simulink model "RLModel"  (R2024b)
settings: Solver=VariableStepAuto  StartTime=0.0  StopTime=Tf  RelTol=1e-3  AbsTol=1e-3  EnableMultiTasking=on
InitFcn:
  | ModelParameters;
values from neighbouring files (symbols this model uses):
  foot_height = 0.05    [ModelParameters.m]
  foot_length = 0.3    [ModelParameters.m]
  foot_width = 0.2    [ModelParameters.m]
  init_height = plane_height/2 + foot_height + shank_height + thigh_height + 0.5*torso_height    (= 1.65)    [ModelParameters.m]
  max_torque = 1000    [ModelParameters.m]
  plane_height = 0.2    [ModelParameters.m]
  shank_height = 0.5    [ModelParameters.m]
  shank_length = 0.2    [ModelParameters.m]
  shank_width = 0.2    [ModelParameters.m]
  thigh_height = 0.5    [ModelParameters.m]
  thigh_length = 0.2    [ModelParameters.m]
  thigh_width = 0.2    [ModelParameters.m]
  torso_height = 1.0    (= 1)    [ModelParameters.m]
  torso_length = 0.2    [ModelParameters.m]
  torso_width = 0.5    [ModelParameters.m]
undefined symbols (not defined in the file or in its folder): X, Y, Z
libraries: sm_lib x53, nesl_utility x32, simulink x2, rllib x1, aerolibconvert2 x1
(part 3 of 3)

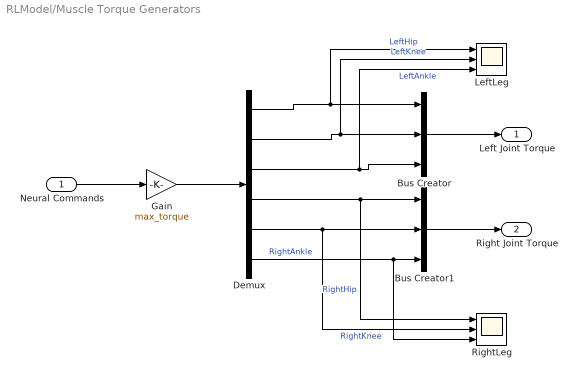
== system RLModel/Muscle Torque Generators ==
  Neural Commands : Inport
  Bus Creator : BusCreator  Inputs=3
  Bus Creator1 : BusCreator  Inputs=3
  Demux : Demux  Outputs=6
  Gain : Gain  Gain=max_torque
  LeftLeg : Scope  NumInputPorts=3
  RightLeg : Scope  NumInputPorts=3
  Left Joint Torque : Outport
  Right Joint Torque : Outport  Port=2
  wires:
  Demux/1 -> LeftLeg/1, Bus Creator/1  "LeftHip"
  Bus Creator/1 -> Left Joint Torque/1
  Bus Creator1/1 -> Right Joint Torque/1
  Demux/2 -> LeftLeg/2, Bus Creator/2  "LeftKnee"
  Demux/3 -> LeftLeg/3, Bus Creator/3  "LeftAnkle"
  Demux/4 -> RightLeg/1, Bus Creator1/1  "RightHip"
  Demux/5 -> Bus Creator1/2, RightLeg/2  "RightKnee"
  Demux/6 -> RightLeg/3, Bus Creator1/3  "RightAnkle"
  Neural Commands/1 -> Gain/1
  Gain/1 -> Demux/1

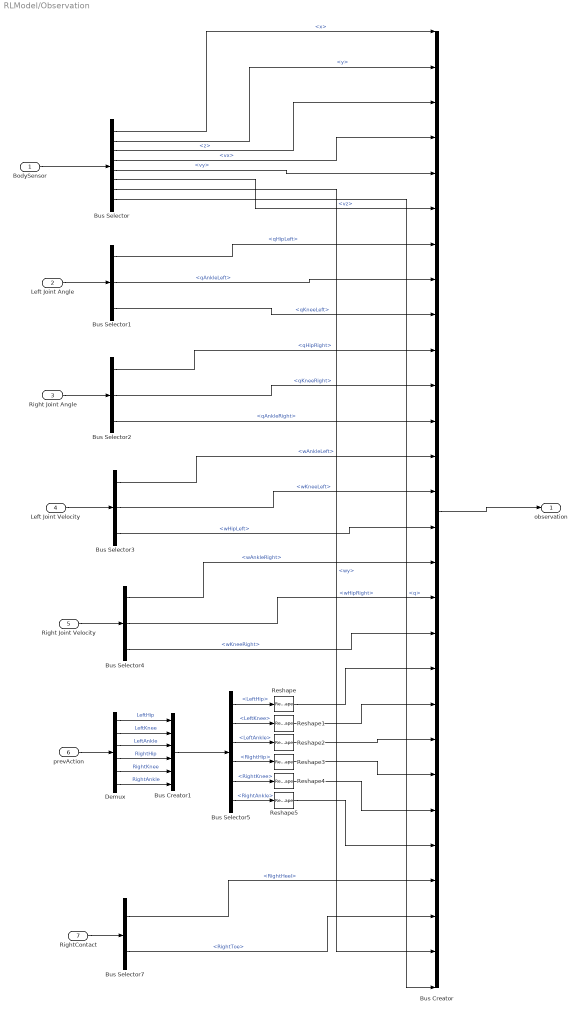
== system RLModel/Observation ==
  BodySensor : Inport
  Left Joint Angle : Inport  Port=2
  Right Joint Angle : Inport  Port=3
  Left Joint Velocity : Inport  Port=4
  Right Joint Velocity : Inport  Port=5
  prevAction : Inport  Port=6
  RightContact : Inport  Port=7
  Bus Creator : BusCreator  Inputs=28
  Bus Creator1 : BusCreator  Inputs=6
  Bus Selector : BusSelector  OutputSignals=x,y,z,vx,vy,vz,wy,q
  Bus Selector1 : BusSelector  OutputSignals=qHipLeft,qAnkleLeft,qKneeLeft
  Bus Selector2 : BusSelector  OutputSignals=qHipRight,qKneeRight,qAnkleRight
  Bus Selector3 : BusSelector  OutputSignals=wAnkleLeft,wKneeLeft,wHipLeft
  Bus Selector4 : BusSelector  OutputSignals=wAnkleRight,wHipRight,wKneeRight
  Bus Selector5 : BusSelector  OutputSignals=LeftHip,LeftKnee,LeftAnkle,RightHip,RightKnee,RightAnkle
  Bus Selector7 : BusSelector  OutputSignals=RightHeel,RightToe
  Demux : Demux  Outputs=6
  Reshape{,1..5} (6 alike) : Reshape  OutputDimensionality=Customize  OutputDimensions=1
  observation : Outport
  wires:
  BodySensor/1 -> Bus Selector/1
  Left Joint Angle/1 -> Bus Selector1/1
  Right Joint Angle/1 -> Bus Selector2/1
  Left Joint Velocity/1 -> Bus Selector3/1
  Right Joint Velocity/1 -> Bus Selector4/1
  Bus Selector/1 -> Bus Creator/1  "<x>"
  Bus Selector/2 -> Bus Creator/2  "<y>"
  Bus Selector/3 -> Bus Creator/3  "<z>"
  Bus Selector/4 -> Bus Creator/4  "<vx>"
  Bus Selector/5 -> Bus Creator/5  "<vy>"
  Bus Selector/6 -> Bus Creator/6  "<vz>"
  Bus Selector1/1 -> Bus Creator/7  "<qHipLeft>"
  Bus Selector1/2 -> Bus Creator/8  "<qAnkleLeft>"
  Bus Selector1/3 -> Bus Creator/9  "<qKneeLeft>"
  Bus Selector2/1 -> Bus Creator/10  "<qHipRight>"
  Bus Selector2/2 -> Bus Creator/11  "<qKneeRight>"
  Bus Selector2/3 -> Bus Creator/12  "<qAnkleRight>"
  Bus Selector3/1 -> Bus Creator/13  "<wAnkleLeft>"
  Bus Selector3/2 -> Bus Creator/14  "<wKneeLeft>"
  Bus Selector3/3 -> Bus Creator/15  "<wHipLeft>"
  Bus Selector4/1 -> Bus Creator/16  "<wAnkleRight>"
  Bus Selector4/2 -> Bus Creator/17  "<wHipRight>"
  Bus Selector4/3 -> Bus Creator/18  "<wKneeRight>"
  Bus Creator/1 -> observation/1
  prevAction/1 -> Demux/1
  Demux/1 -> Bus Creator1/1  "LeftHip"
  Demux/2 -> Bus Creator1/2  "LeftKnee"
  Demux/3 -> Bus Creator1/3  "LeftAnkle"
  Demux/4 -> Bus Creator1/4  "RightHip"
  Demux/5 -> Bus Creator1/5  "RightKnee"
  Demux/6 -> Bus Creator1/6  "RightAnkle"
  Bus Creator1/1 -> Bus Selector5/1
  Bus Selector5/1 -> Reshape/1  "<LeftHip>"
  Reshape/1 -> Bus Creator/19
  Bus Selector5/2 -> Reshape1/1  "<LeftKnee>"
  Bus Selector5/3 -> Reshape2/1  "<LeftAnkle>"
  Bus Selector5/4 -> Reshape3/1  "<RightHip>"
  Bus Selector5/5 -> Reshape4/1  "<RightKnee>"
  Bus Selector5/6 -> Reshape5/1  "<RightAnkle>"
  Reshape1/1 -> Bus Creator/20
  Reshape2/1 -> Bus Creator/21
  Reshape3/1 -> Bus Creator/22
  Reshape4/1 -> Bus Creator/23
  Reshape5/1 -> Bus Creator/24
  RightContact/1 -> Bus Selector7/1
  Bus Selector7/1 -> Bus Creator/25  "<RightHeel>"
  Bus Selector7/2 -> Bus Creator/26  "<RightToe>"
  Bus Selector/7 -> Bus Creator/27  "<wy>"
  Bus Selector/8 -> Bus Creator/28  "<q>"

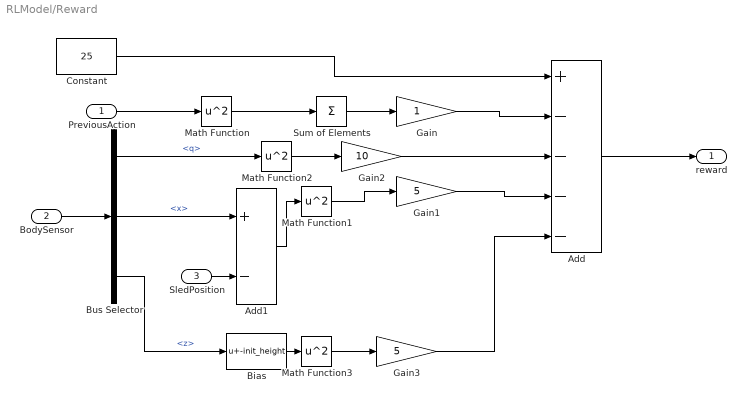
== system RLModel/Reward ==
  PreviousAction : Inport
  BodySensor : Inport  Port=2
  SledPosition : Inport  Port=3
  Add : Sum  Inputs=+----
  Add1 : Sum  Inputs=+-
  Bias : Bias  Bias=-init_height  SaturateOnIntegerOverflow=off
  Bus Selector : BusSelector  OutputSignals=q,x,z
  Constant : Constant  Value=25
  Gain : Gain
  Gain1 : Gain  Gain=5
  Gain2 : Gain  Gain=10
  Gain3 : Gain  Gain=5
  Math Function{,1..3} (4 alike) : Math  Operator=square
  Sum of Elements : Sum  Inputs=+
  reward : Outport
  wires:
  PreviousAction/1 -> Math Function/1
  Math Function/1 -> Sum of Elements/1
  Sum of Elements/1 -> Gain/1
  Add/1 -> reward/1
  BodySensor/1 -> Bus Selector/1
  Bus Selector/2 -> Add1/1  "<x>"
  SledPosition/1 -> Add1/2
  Add1/1 -> Math Function1/1
  Math Function1/1 -> Gain1/1
  Bus Selector/1 -> Math Function2/1  "<q>"
  Math Function2/1 -> Gain2/1
  Bias/1 -> Math Function3/1
  Math Function3/1 -> Gain3/1
  Bus Selector/3 -> Bias/1  "<z>"
  Gain/1 -> Add/2
  Gain2/1 -> Add/3
  Gain1/1 -> Add/4
  Gain3/1 -> Add/5
  Constant/1 -> Add/1

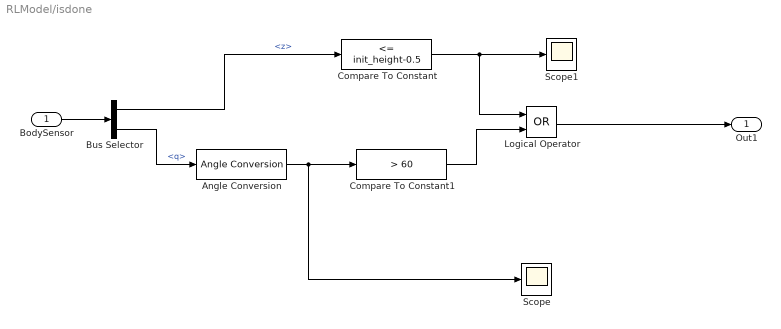
== system RLModel/isdone ==
  BodySensor : Inport
  Angle Conversion : aerolibconvert2/Angle Conversion  IU=rad  OU=deg
  Bus Selector : BusSelector  OutputSignals=z,q
  Compare To Constant : simulink/Logic and Bit Operations/Compare To Constant  relop=<=  const=init_height-0.5  OutDataTypeStr=boolean
  Compare To Constant1 : simulink/Logic and Bit Operations/Compare To Constant  relop=>  const=60  OutDataTypeStr=boolean
  Logical Operator : Logic  Operator=OR  AllPortsSameDT=off  OutDataTypeStr=boolean
  Scope : Scope
  Scope1 : Scope
  Out1 : Outport
  wires:
  BodySensor/1 -> Bus Selector/1
  Bus Selector/1 -> Compare To Constant/1  "<z>"
  Bus Selector/2 -> Angle Conversion/1  "<q>"
  Compare To Constant1/1 -> Logical Operator/2
  Compare To Constant/1 -> Scope1/1, Logical Operator/1
  Logical Operator/1 -> Out1/1
  Angle Conversion/1 -> Scope/1, Compare To Constant1/1

== matlab function RLModel/MATLAB Function ==
  data: t input; x output; a input; x_max input
function x = fcn(t,a,x_max)

t1 = sqrt((x_max / 2) * 2 / a);   % Time to halfway point
t_total = 2 * t1;                 % Total time of motion


if t < t1
    x = 0.5*a*(t^2);
elseif t >= t1 && t <= t_total
    td = t-t1;
    v_max = a*t1;
    x = (x_max/2) + v_max*td - 0.5*a*(td^2);
else
    x = x_max;
end

end
